simulink model "uavsim_trim"  (R2022a)
settings: Solver=VariableStepAuto  StartTime=0.0  StopTime=10.0  RelTol=1e-3
undefined symbols (not defined in the file or in its folder): forces_moments, UAV
settings Model: Creator=21024906d  LastModifiedBy=heiwong
settings SolverCC: AlgebraicLoopSolver=TrustRegion
settings DebuggingCC: UnconnectedInputMsg=warning  UnconnectedOutputMsg=warning  UnconnectedLineMsg=warning  SFMachineParentedDataDiag=warning

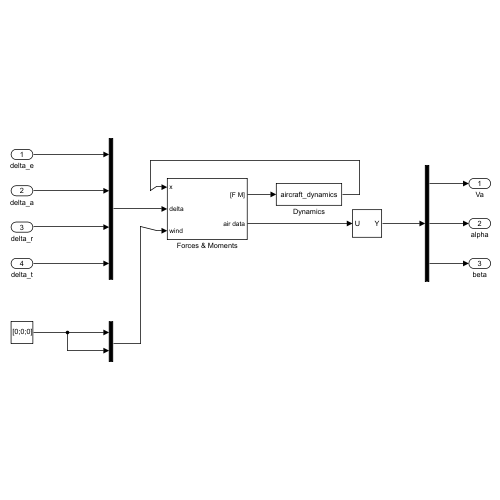
[thumbnail: Simulink's stored preview of the top-level diagram]
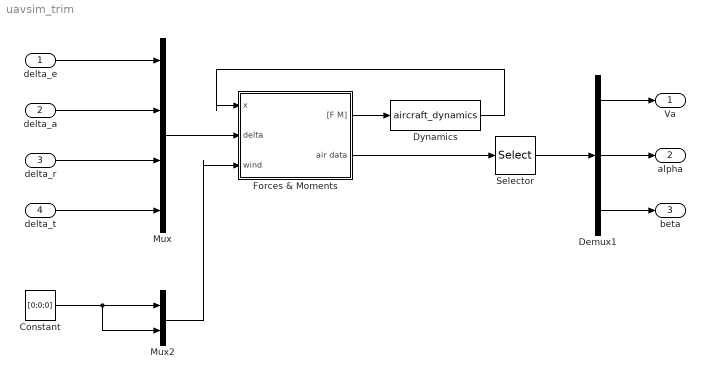
== system uavsim_trim ==
  delta_e : Inport
  delta_a : Inport  Port=2
  delta_r : Inport  Port=3
  delta_t : Inport  Port=4
  Constant : Constant  Value=[0;0;0]
  Demux1 : Demux  Outputs=3
  Dynamics : S-Function  FunctionName=aircraft_dynamics  Parameters=UAV  SFunctionDeploymentMode=off  EnableBusSupport=off
  Forces & Moments : Subsystem
  Mux : Mux
  Mux2 : Mux  Inputs=2
  Selector : Selector  InputPortWidth=6  IndexOptions=Index vector (dialog)  Indices=[1 2 3]  OutputSizes=1
  Va : Outport
  alpha : Outport  Port=2
  beta : Outport  Port=3
  wires:
  Mux/1 -> Forces & Moments/2(delta)
  delta_e/1 -> Mux/1
  delta_a/1 -> Mux/2
  delta_r/1 -> Mux/3
  delta_t/1 -> Mux/4
  Forces & Moments/1("[F M]") -> Dynamics/1
  Demux1/3 -> beta/1
  Demux1/2 -> alpha/1
  Demux1/1 -> Va/1
  Forces & Moments/2(air data) -> Selector/1
  Dynamics/1 -> Forces & Moments/1(x)
  Constant/1 -> Mux2/1, Mux2/2
  Mux2/1 -> Forces & Moments/3(wind)
  Selector/1 -> Demux1/1

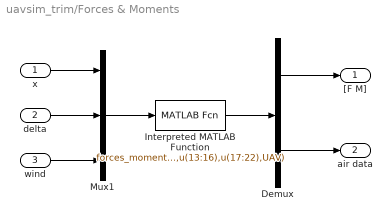
== system uavsim_trim/Forces & Moments ==
  x : Inport
  delta : Inport  Port=2
  wind : Inport  Port=3
  Demux : Demux  Outputs=[6;6]
  Interpreted MATLAB Function : MATLABFcn  MATLABFcn=forces_moments(u(1:12),u(13:16),u(17:22),UAV)  OutputDimensions=12
  Mux1 : Mux  Inputs=3
  "[F M]" : Outport
  air data : Outport  Port=2
  wires:
  x/1 -> Mux1/1
  Mux1/1 -> Interpreted MATLAB Function/1
  wind/1 -> Mux1/3
  Demux/1 -> "[F M]"/1
  delta/1 -> Mux1/2
  Interpreted MATLAB Function/1 -> Demux/1
  Demux/2 -> air data/1
